simulink model "RexProblemSet2"  (R2020a)
settings: Solver=VariableStepAuto  StartTime=0.0  StopTime=10.0  RelTol=1e-3
undefined symbols (not defined in the file): gray
libraries: commutil2 x6, dspindex x4, visiontextngfix x2, visionsources x2
settings Model: Creator=23RexL  LastModifiedBy=23RexL

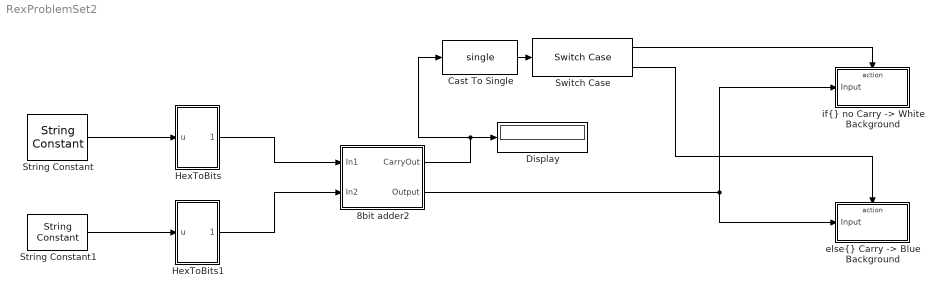
== system RexProblemSet2 ==
  8bit adder2 : Subsystem
  Cast To Single : DataTypeConversion  OutDataTypeStr=single
  Display : Display
  HexToBits : Subsystem
  HexToBits1 : Subsystem
  String Constant : StringConstant  String="\"FF\""
  String Constant1 : StringConstant  String="\"01\""
  Switch Case : SwitchCase  CaseConditions={0,1}  ShowDefaultCase=off  ZeroCross=off
  "else{} Carry -> Blue Background" : Subsystem  TreatAsAtomicUnit=on
  "if{} no Carry -> White Background" : Subsystem  TreatAsAtomicUnit=on
  wires:
  HexToBits/1(Out1) -> 8bit adder2/1(In1)
  String Constant1/1 -> HexToBits1/1(u)
  HexToBits1/1(Out1) -> 8bit adder2/2(In2)
  8bit adder2/1(CarryOut) -> Display/1, Cast To Single/1
  String Constant/1 -> HexToBits/1(u)
  Switch Case/2 -> "else{} Carry -> Blue Background"/Action
  Switch Case/1 -> "if{} no Carry -> White Background"/Action
  Cast To Single/1 -> Switch Case/1
  8bit adder2/2(Output) -> "if{} no Carry -> White Background"/1(Input), "else{} Carry -> Blue Background"/1(Input)

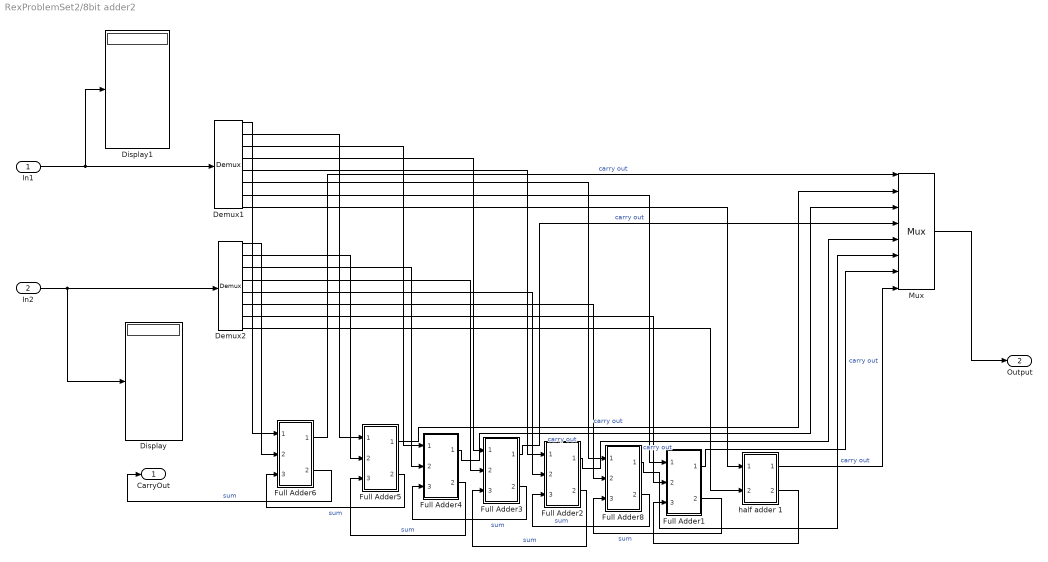
== system RexProblemSet2/8bit adder2 ==
  In1 : Inport
  In2 : Inport  Port=2
  Demux1 : Demux  Outputs=8
  Demux2 : Demux  Outputs=8
  Display : Display
  Display1 : Display
  Full Adder1 : Subsystem
  Full Adder2 : Subsystem
  Full Adder3 : Subsystem
  Full Adder4 : Subsystem
  Full Adder5 : Subsystem
  Full Adder6 : Subsystem
  Full Adder8 : Subsystem
  Mux : Mux  Inputs=8
  half adder 1 : Subsystem
  CarryOut : Outport
  Output : Outport  Port=2
  wires:
  Demux2/6 -> Full Adder8/2(Input1)
  Demux1/4 -> Full Adder3/1(Input)
  Demux2/4 -> Full Adder3/2(Input1)
  Demux2/8 -> half adder 1/2(Input2)
  Full Adder4/2(Output) -> Full Adder5/3(Input2)  "sum"
  Demux2/7 -> Full Adder1/2(Input1)
  Full Adder8/2(Output) -> Full Adder2/3(Input2)  "sum"
  Demux2/1 -> Full Adder6/2(Input1)
  Demux1/8 -> half adder 1/1(In1)
  Full Adder1/2(Output) -> Full Adder8/3(Input2)  "sum"
  In2/1 -> Display/1, Demux2/1
  Full Adder8/1(Output1) -> Mux/6  "carry out"
  Full Adder6/1(Output1) -> Mux/1  "carry out"
  Full Adder4/1(Output1) -> Mux/3  "carry out"
  Demux2/2 -> Full Adder5/2(Input1)
  Demux1/3 -> Full Adder4/1(Input)
  Full Adder5/1(Output1) -> Mux/2  "carry out"
  Demux2/3 -> Full Adder4/2(Input1)
  Full Adder3/1(Output1) -> Mux/4  "carry out"
  Full Adder3/2(Output) -> Full Adder4/3(Input2)  "sum"
  In1/1 -> Demux1/1, Display1/1
  Demux2/5 -> Full Adder2/2(Input1)
  Full Adder2/2(Output) -> Full Adder3/3(Input2)  "sum"
  half adder 1/2(Out2) -> Full Adder1/3(Input2)
  Full Adder2/1(Output1) -> Mux/5  "carry out"
  Demux1/5 -> Full Adder2/1(Input)
  Demux1/2 -> Full Adder5/1(Input)
  Full Adder5/2(Output) -> Full Adder6/3(Input2)  "sum"
  Demux1/1 -> Full Adder6/1(Input)
  Full Adder1/1(Output1) -> Mux/7  "carry out"
  half adder 1/1(Out1) -> Mux/8
  Demux1/7 -> Full Adder1/1(Input)
  Demux1/6 -> Full Adder8/1(Input)
  Mux/1 -> Output/1
  Full Adder6/2(Output) -> CarryOut/1  "sum"

== system RexProblemSet2/HexToBits ==
  u : Inport
  Integer to Bit Converter : commutil2/Integer to Bit Converter  nbits=8  signedInputValues=Unsigned  bitOrder=MSB first  outDtype=Inherit via internal rule
  MATLAB Function : MATLAB Function  TreatAsAtomicUnit=on
  Out1 : Outport
  wires:
  MATLAB Function/1(y) -> Integer to Bit Converter/1
  u/1 -> MATLAB Function/1(u)
  Integer to Bit Converter/1 -> Out1/1

== system RexProblemSet2/HexToBits1 ==
  u : Inport
  Integer to Bit Converter : commutil2/Integer to Bit Converter  nbits=8  signedInputValues=Unsigned  bitOrder=MSB first  outDtype=Inherit via internal rule
  MATLAB Function : MATLAB Function  TreatAsAtomicUnit=on
  Out1 : Outport
  wires:
  MATLAB Function/1(y) -> Integer to Bit Converter/1
  u/1 -> MATLAB Function/1(u)
  Integer to Bit Converter/1 -> Out1/1

== system RexProblemSet2/else{} Carry -> Blue Background ==
  Input : Inport
  Action Port : ActionPort  ActionPortLabel=case [ 1 ]:
  "else{} Carry -> Blue Background" : Subsystem
  wires:
  Input/1 -> "else{} Carry -> Blue Background"/1(Input1)

== system RexProblemSet2/if{} no Carry -> White Background ==
  Input : Inport
  Action Port : ActionPort  PropagateVarSize=During execution  ActionPortLabel=case [ 0 ]:
  "if{} no Carry -> White Background" : Subsystem
  wires:
  Input/1 -> "if{} no Carry -> White Background"/1(Input)

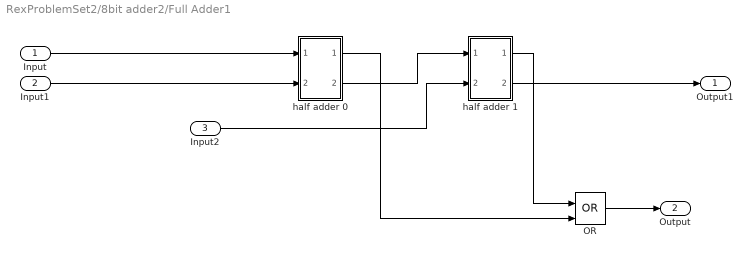
== system RexProblemSet2/8bit adder2/Full Adder1 ==
  Input : Inport
  Input1 : Inport  Port=2
  Input2 : Inport  Port=3
  OR : Logic  Operator=OR  IconShape=distinctive  AllPortsSameDT=off  OutDataTypeStr=boolean
  half adder 0 : Subsystem
  half adder 1 : Subsystem
  Output1 : Outport
  Output : Outport  Port=2
  wires:
  half adder 0/1(Out1) -> OR/2
  Input/1 -> half adder 0/1(Input)
  Input1/1 -> half adder 0/2(Input1)
  half adder 0/2(Out2) -> half adder 1/1(In1)
  half adder 1/1(Out1) -> OR/1
  OR/1 -> Output/1
  half adder 1/2(Output1) -> Output1/1
  Input2/1 -> half adder 1/2(Input2)

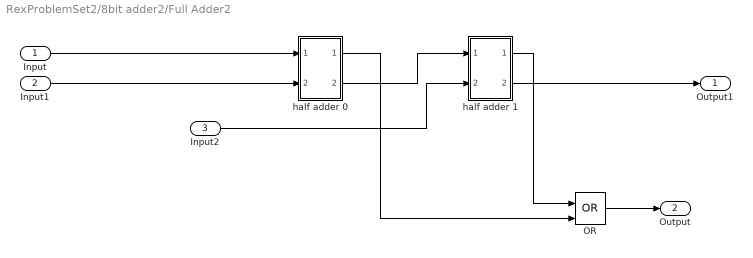
== system RexProblemSet2/8bit adder2/Full Adder2 ==
  Input : Inport
  Input1 : Inport  Port=2
  Input2 : Inport  Port=3
  OR : Logic  Operator=OR  IconShape=distinctive  AllPortsSameDT=off  OutDataTypeStr=boolean
  half adder 0 : Subsystem
  half adder 1 : Subsystem
  Output1 : Outport
  Output : Outport  Port=2
  wires:
  half adder 0/1(Out1) -> OR/2
  Input/1 -> half adder 0/1(Input)
  Input1/1 -> half adder 0/2(Input1)
  half adder 0/2(Out2) -> half adder 1/1(In1)
  half adder 1/1(Out1) -> OR/1
  OR/1 -> Output/1
  half adder 1/2(Output1) -> Output1/1
  Input2/1 -> half adder 1/2(Input2)

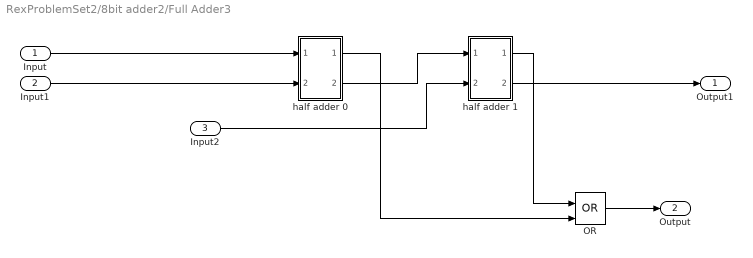
== system RexProblemSet2/8bit adder2/Full Adder3 ==
  Input : Inport
  Input1 : Inport  Port=2
  Input2 : Inport  Port=3
  OR : Logic  Operator=OR  IconShape=distinctive  AllPortsSameDT=off  OutDataTypeStr=boolean
  half adder 0 : Subsystem
  half adder 1 : Subsystem
  Output1 : Outport
  Output : Outport  Port=2
  wires:
  half adder 0/1(Out1) -> OR/2
  Input/1 -> half adder 0/1(Input)
  Input1/1 -> half adder 0/2(Input1)
  half adder 0/2(Out2) -> half adder 1/1(In1)
  half adder 1/1(Out1) -> OR/1
  OR/1 -> Output/1
  half adder 1/2(Output1) -> Output1/1
  Input2/1 -> half adder 1/2(Input2)

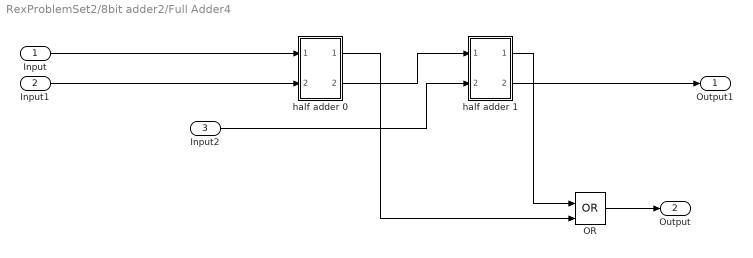
== system RexProblemSet2/8bit adder2/Full Adder4 ==
  Input : Inport
  Input1 : Inport  Port=2
  Input2 : Inport  Port=3
  OR : Logic  Operator=OR  IconShape=distinctive  AllPortsSameDT=off  OutDataTypeStr=boolean
  half adder 0 : Subsystem
  half adder 1 : Subsystem
  Output1 : Outport
  Output : Outport  Port=2
  wires:
  half adder 0/1(Out1) -> OR/2
  Input/1 -> half adder 0/1(Input)
  Input1/1 -> half adder 0/2(Input1)
  half adder 0/2(Out2) -> half adder 1/1(In1)
  half adder 1/1(Out1) -> OR/1
  OR/1 -> Output/1
  half adder 1/2(Output1) -> Output1/1
  Input2/1 -> half adder 1/2(Input2)

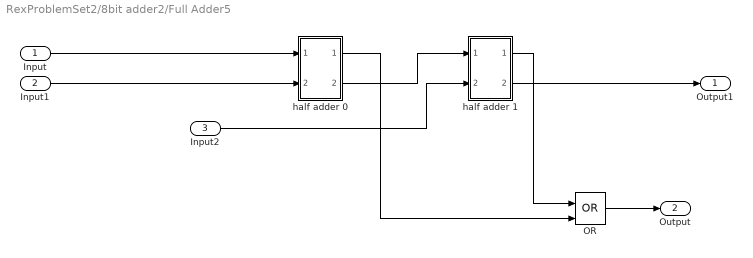
== system RexProblemSet2/8bit adder2/Full Adder5 ==
  Input : Inport
  Input1 : Inport  Port=2
  Input2 : Inport  Port=3
  OR : Logic  Operator=OR  IconShape=distinctive  AllPortsSameDT=off  OutDataTypeStr=boolean
  half adder 0 : Subsystem
  half adder 1 : Subsystem
  Output1 : Outport
  Output : Outport  Port=2
  wires:
  half adder 0/1(Out1) -> OR/2
  Input/1 -> half adder 0/1(Input)
  Input1/1 -> half adder 0/2(Input1)
  half adder 0/2(Out2) -> half adder 1/1(In1)
  half adder 1/1(Out1) -> OR/1
  OR/1 -> Output/1
  half adder 1/2(Output1) -> Output1/1
  Input2/1 -> half adder 1/2(Input2)

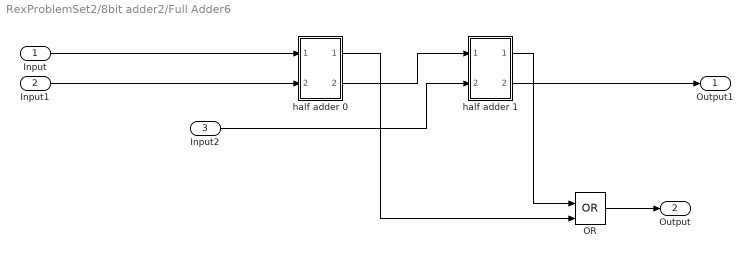
== system RexProblemSet2/8bit adder2/Full Adder6 ==
  Input : Inport
  Input1 : Inport  Port=2
  Input2 : Inport  Port=3
  OR : Logic  Operator=OR  IconShape=distinctive  AllPortsSameDT=off  OutDataTypeStr=boolean
  half adder 0 : Subsystem
  half adder 1 : Subsystem
  Output1 : Outport
  Output : Outport  Port=2
  wires:
  half adder 0/1(Out1) -> OR/2
  Input/1 -> half adder 0/1(Input)
  Input1/1 -> half adder 0/2(Input1)
  half adder 0/2(Out2) -> half adder 1/1(In1)
  half adder 1/1(Out1) -> OR/1
  OR/1 -> Output/1
  half adder 1/2(Output1) -> Output1/1
  Input2/1 -> half adder 1/2(Input2)

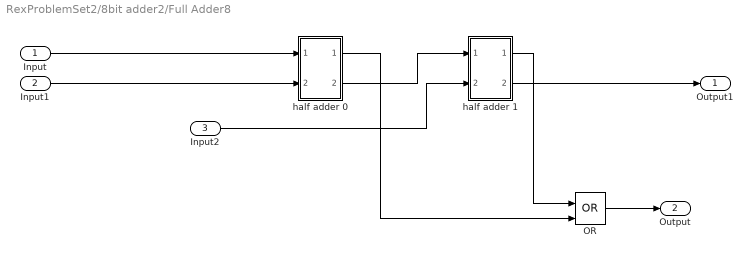
== system RexProblemSet2/8bit adder2/Full Adder8 ==
  Input : Inport
  Input1 : Inport  Port=2
  Input2 : Inport  Port=3
  OR : Logic  Operator=OR  IconShape=distinctive  AllPortsSameDT=off  OutDataTypeStr=boolean
  half adder 0 : Subsystem
  half adder 1 : Subsystem
  Output1 : Outport
  Output : Outport  Port=2
  wires:
  half adder 0/1(Out1) -> OR/2
  Input/1 -> half adder 0/1(Input)
  Input1/1 -> half adder 0/2(Input1)
  half adder 0/2(Out2) -> half adder 1/1(In1)
  half adder 1/1(Out1) -> OR/1
  OR/1 -> Output/1
  half adder 1/2(Output1) -> Output1/1
  Input2/1 -> half adder 1/2(Input2)

== system RexProblemSet2/8bit adder2/half adder 1 ==
  In1 : Inport
  Input2 : Inport  Port=2
  NAND : Logic  IconShape=distinctive  AllPortsSameDT=off  OutDataTypeStr=boolean
  XOR : Logic  Operator=XOR  IconShape=distinctive  AllPortsSameDT=off  OutDataTypeStr=boolean
  Out1 : Outport
  Out2 : Outport  Port=2
  wires:
  Input2/1 -> NAND/2, XOR/2
  In1/1 -> NAND/1, XOR/1
  NAND/1 -> Out2/1
  XOR/1 -> Out1/1

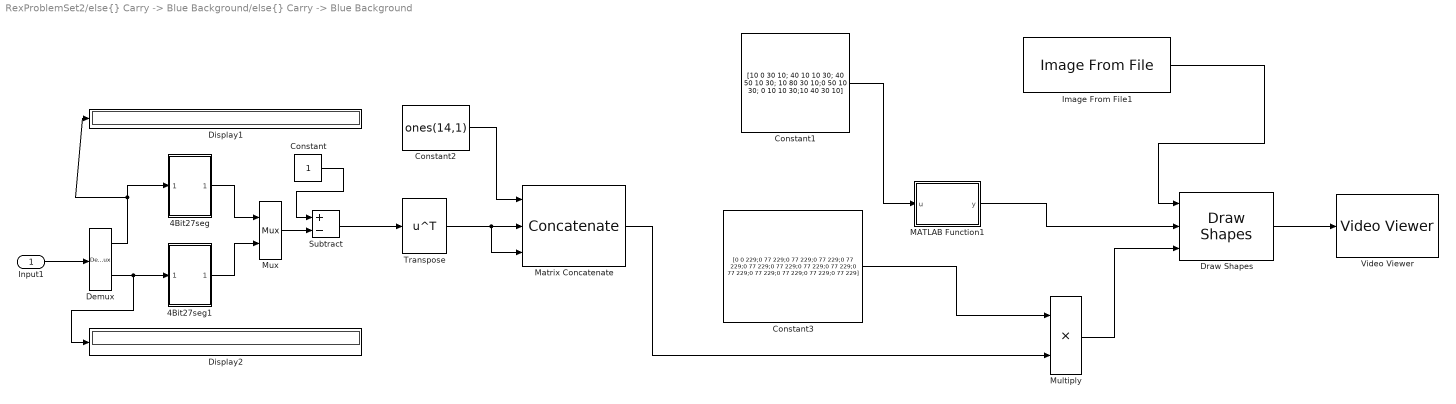
== system RexProblemSet2/else{} Carry -> Blue Background/else{} Carry -> Blue Background ==
  Input1 : Inport
  4Bit27seg : Subsystem
  4Bit27seg1 : Subsystem
  Constant : Constant
  Constant1 : Constant  Value="[10 0  30 10; 40 10 10 30; 40 50 10 30; 10 80 30 10;0 50 10 30; 0 10 10 30;10 40 30 10]"  VectorParams1D=off
  Constant2 : Constant  Value=ones(14,1)
  Constant3 : Constant  Value=[0 0 229;0 77 229;0 77 229;0 77 229;0 77 229;0 77 229;0 77 229;0 77 229;0 77 229;0 77 229;0 77 229;0 77 229;0 77 229;0 77 229]  VectorParams1D=off
  Demux : Demux  Outputs=2
  Display1 : Display
  Display2 : Display
  Draw Shapes : visiontextngfix/Draw Shapes  shape=Rectangles  fill=on  lineWidth=1  fillClrSource=Input port  display=Black  intensity=200  color=[200 255 100]  opacity=0.6  viewport=Entire image  antialiasing=off  inType=Obsolete  imagePorts=One multidimensional signal  roundingMode=Floor  overflowMode=off  memoryMode=Specify word length  memoryWordLength=16  prodOutputMode=Binary point scaling  prodOutputWordLength=32  prodOutputFracLength=14  memoryFracLength=14
  Image From File1 : visionsources/Image From File  Tag=vipblks_nd  FileName=C:\Users\23rexl\Desktop\Rex ProblemSet 2\BlueBackground.jpg  Ts=inf  imagePorts=One multidimensional signal  OutPortLabels=R|G|B  ImageDataType=double  sdImageDataType=uint(8)  Signed=on  WordLength=16  FractionLengthMode=User-defined  FractionLength=15
      link override Constant1: Value=ImageValue
  MATLAB Function1 : MATLAB Function  TreatAsAtomicUnit=on
  Matrix Concatenate : Concatenate  NumInputs=3  Mode=Multidimensional array  ConcatenateDimension=2
  Multiply : Product
  Mux : Mux  Inputs=2
  Subtract : Sum  Inputs=+-
  Transpose : Math  Operator=transpose  SaturateOnIntegerOverflow=on
  Video Viewer : VideoViewer  colormapValue=gray(256)  FigPos=[810.6 762 480.8 371.2]
  wires:
  Mux/1 -> Subtract/2
  Constant2/1 -> Matrix Concatenate/1
  Matrix Concatenate/1 -> Multiply/2
  Multiply/1 -> Draw Shapes/3
  Constant3/1 -> Multiply/1
  Demux/1 -> 4Bit27seg/1(Input), Display1/1
  Subtract/1 -> Transpose/1
  Draw Shapes/1 -> Video Viewer/1
  4Bit27seg1/1(Output) -> Mux/2
  Demux/2 -> Display2/1, 4Bit27seg1/1(Input)
  Constant1/1 -> MATLAB Function1/1(u)
  4Bit27seg/1(Output) -> Mux/1
  Constant/1 -> Subtract/1
  Image From File1/1 -> Draw Shapes/1
  MATLAB Function1/1(y) -> Draw Shapes/2
  Transpose/1 -> Matrix Concatenate/3, Matrix Concatenate/2
  Input1/1 -> Demux/1

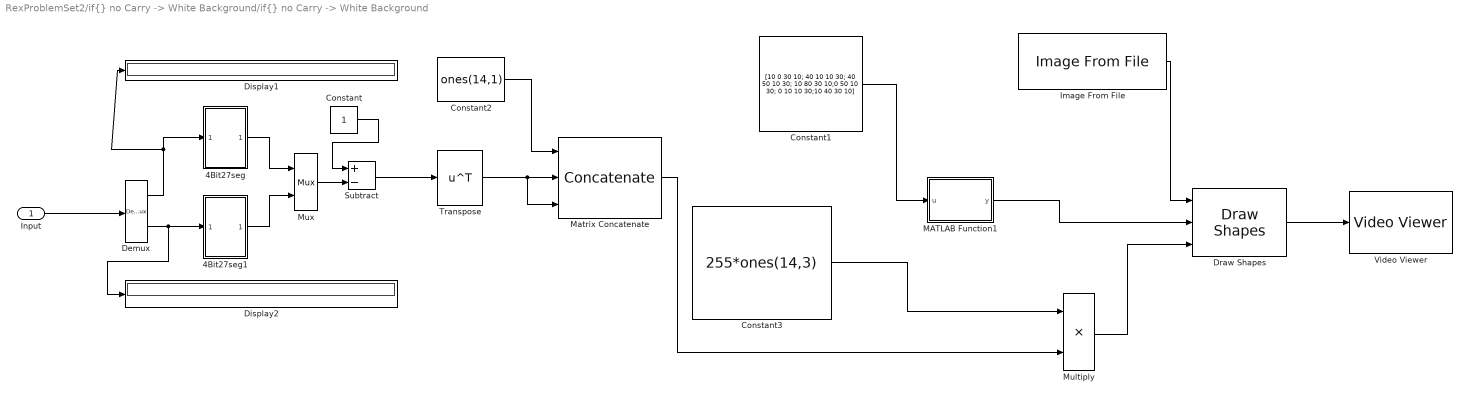
== system RexProblemSet2/if{} no Carry -> White Background/if{} no Carry -> White Background ==
  Input : Inport
  4Bit27seg : Subsystem
  4Bit27seg1 : Subsystem
  Constant : Constant
  Constant1 : Constant  Value="[10 0  30 10; 40 10 10 30; 40 50 10 30; 10 80 30 10;0 50 10 30; 0 10 10 30;10 40 30 10]"  VectorParams1D=off
  Constant2 : Constant  Value=ones(14,1)
  Constant3 : Constant  Value=255*ones(14,3)
  Demux : Demux  Outputs=2
  Display1 : Display
  Display2 : Display
  Draw Shapes : visiontextngfix/Draw Shapes  shape=Rectangles  fill=on  lineWidth=1  fillClrSource=Input port  display=Black  intensity=200  color=[200 255 100]  opacity=0.6  viewport=Entire image  antialiasing=off  inType=Obsolete  imagePorts=One multidimensional signal  roundingMode=Floor  overflowMode=off  memoryMode=Specify word length  memoryWordLength=16  prodOutputMode=Binary point scaling  prodOutputWordLength=32  prodOutputFracLength=14  memoryFracLength=14
  Image From File : visionsources/Image From File  Tag=vipblks_nd  FileName=C:\Users\23rexl\Desktop\Rex ProblemSet 2\WhiteBackground (1).png  Ts=inf  imagePorts=One multidimensional signal  OutPortLabels=R|G|B  ImageDataType=double  sdImageDataType=uint(8)  Signed=on  WordLength=16  FractionLengthMode=User-defined  FractionLength=15
      link override Constant1: Value=ImageValue
  MATLAB Function1 : MATLAB Function  TreatAsAtomicUnit=on
  Matrix Concatenate : Concatenate  NumInputs=3  Mode=Multidimensional array  ConcatenateDimension=2
  Multiply : Product
  Mux : Mux  Inputs=2
  Subtract : Sum  Inputs=+-
  Transpose : Math  Operator=transpose  SaturateOnIntegerOverflow=on
  Video Viewer : VideoViewer  colormapValue=gray(256)  FigPos=[117.8 924.4 648 477.6]
  wires:
  Mux/1 -> Subtract/2
  Constant2/1 -> Matrix Concatenate/1
  Matrix Concatenate/1 -> Multiply/2
  Multiply/1 -> Draw Shapes/3
  Constant3/1 -> Multiply/1
  Demux/1 -> 4Bit27seg/1(Input), Display1/1
  Subtract/1 -> Transpose/1
  Draw Shapes/1 -> Video Viewer/1
  4Bit27seg1/1(Output) -> Mux/2
  Demux/2 -> Display2/1, 4Bit27seg1/1(Input)
  Constant1/1 -> MATLAB Function1/1(u)
  4Bit27seg/1(Output) -> Mux/1
  Constant/1 -> Subtract/1
  Image From File/1 -> Draw Shapes/1
  MATLAB Function1/1(y) -> Draw Shapes/2
  Transpose/1 -> Matrix Concatenate/3, Matrix Concatenate/2
  Input/1 -> Demux/1

== system RexProblemSet2/8bit adder2/Full Adder1/half adder 0 ==
  Input : Inport
  Input1 : Inport  Port=2
  XOR : Logic  Operator=XOR  IconShape=distinctive  AllPortsSameDT=off  OutDataTypeStr=boolean
  and : Logic  IconShape=distinctive  AllPortsSameDT=off  OutDataTypeStr=boolean
  Out1 : Outport
  Out2 : Outport  Port=2
  wires:
  Input1/1 -> and/2, XOR/2
  Input/1 -> and/1, XOR/1
  and/1 -> Out1/1
  XOR/1 -> Out2/1

== system RexProblemSet2/8bit adder2/Full Adder1/half adder 1 ==
  In1 : Inport
  Input2 : Inport  Port=2
  AND : Logic  IconShape=distinctive  AllPortsSameDT=off  OutDataTypeStr=boolean
  XOR : Logic  Operator=XOR  IconShape=distinctive  AllPortsSameDT=off  OutDataTypeStr=boolean
  Out1 : Outport
  Output1 : Outport  Port=2
  wires:
  Input2/1 -> AND/2, XOR/2
  In1/1 -> AND/1, XOR/1
  AND/1 -> Out1/1
  XOR/1 -> Output1/1

== system RexProblemSet2/8bit adder2/Full Adder2/half adder 0 ==
  Input : Inport
  Input1 : Inport  Port=2
  XOR : Logic  Operator=XOR  IconShape=distinctive  AllPortsSameDT=off  OutDataTypeStr=boolean
  and : Logic  IconShape=distinctive  AllPortsSameDT=off  OutDataTypeStr=boolean
  Out1 : Outport
  Out2 : Outport  Port=2
  wires:
  Input1/1 -> and/2, XOR/2
  Input/1 -> and/1, XOR/1
  and/1 -> Out1/1
  XOR/1 -> Out2/1

== system RexProblemSet2/8bit adder2/Full Adder2/half adder 1 ==
  In1 : Inport
  Input2 : Inport  Port=2
  AND : Logic  IconShape=distinctive  AllPortsSameDT=off  OutDataTypeStr=boolean
  XOR : Logic  Operator=XOR  IconShape=distinctive  AllPortsSameDT=off  OutDataTypeStr=boolean
  Out1 : Outport
  Output1 : Outport  Port=2
  wires:
  Input2/1 -> AND/2, XOR/2
  In1/1 -> AND/1, XOR/1
  AND/1 -> Out1/1
  XOR/1 -> Output1/1

== system RexProblemSet2/8bit adder2/Full Adder3/half adder 0 ==
  Input : Inport
  Input1 : Inport  Port=2
  XOR : Logic  Operator=XOR  IconShape=distinctive  AllPortsSameDT=off  OutDataTypeStr=boolean
  and : Logic  IconShape=distinctive  AllPortsSameDT=off  OutDataTypeStr=boolean
  Out1 : Outport
  Out2 : Outport  Port=2
  wires:
  Input1/1 -> and/2, XOR/2
  Input/1 -> and/1, XOR/1
  and/1 -> Out1/1
  XOR/1 -> Out2/1

== system RexProblemSet2/8bit adder2/Full Adder3/half adder 1 ==
  In1 : Inport
  Input2 : Inport  Port=2
  AND : Logic  IconShape=distinctive  AllPortsSameDT=off  OutDataTypeStr=boolean
  XOR : Logic  Operator=XOR  IconShape=distinctive  AllPortsSameDT=off  OutDataTypeStr=boolean
  Out1 : Outport
  Output1 : Outport  Port=2
  wires:
  Input2/1 -> AND/2, XOR/2
  In1/1 -> AND/1, XOR/1
  AND/1 -> Out1/1
  XOR/1 -> Output1/1

== system RexProblemSet2/8bit adder2/Full Adder4/half adder 0 ==
  Input : Inport
  Input1 : Inport  Port=2
  XOR : Logic  Operator=XOR  IconShape=distinctive  AllPortsSameDT=off  OutDataTypeStr=boolean
  and : Logic  IconShape=distinctive  AllPortsSameDT=off  OutDataTypeStr=boolean
  Out1 : Outport
  Out2 : Outport  Port=2
  wires:
  Input1/1 -> and/2, XOR/2
  Input/1 -> and/1, XOR/1
  and/1 -> Out1/1
  XOR/1 -> Out2/1

== system RexProblemSet2/8bit adder2/Full Adder4/half adder 1 ==
  In1 : Inport
  Input2 : Inport  Port=2
  AND : Logic  IconShape=distinctive  AllPortsSameDT=off  OutDataTypeStr=boolean
  XOR : Logic  Operator=XOR  IconShape=distinctive  AllPortsSameDT=off  OutDataTypeStr=boolean
  Out1 : Outport
  Output1 : Outport  Port=2
  wires:
  Input2/1 -> AND/2, XOR/2
  In1/1 -> AND/1, XOR/1
  AND/1 -> Out1/1
  XOR/1 -> Output1/1

== system RexProblemSet2/8bit adder2/Full Adder5/half adder 0 ==
  Input : Inport
  Input1 : Inport  Port=2
  XOR : Logic  Operator=XOR  IconShape=distinctive  AllPortsSameDT=off  OutDataTypeStr=boolean
  and : Logic  IconShape=distinctive  AllPortsSameDT=off  OutDataTypeStr=boolean
  Out1 : Outport
  Out2 : Outport  Port=2
  wires:
  Input1/1 -> and/2, XOR/2
  Input/1 -> and/1, XOR/1
  and/1 -> Out1/1
  XOR/1 -> Out2/1

== system RexProblemSet2/8bit adder2/Full Adder5/half adder 1 ==
  In1 : Inport
  Input2 : Inport  Port=2
  AND : Logic  IconShape=distinctive  AllPortsSameDT=off  OutDataTypeStr=boolean
  XOR : Logic  Operator=XOR  IconShape=distinctive  AllPortsSameDT=off  OutDataTypeStr=boolean
  Out1 : Outport
  Output1 : Outport  Port=2
  wires:
  Input2/1 -> AND/2, XOR/2
  In1/1 -> AND/1, XOR/1
  AND/1 -> Out1/1
  XOR/1 -> Output1/1

== system RexProblemSet2/8bit adder2/Full Adder6/half adder 0 ==
  Input : Inport
  Input1 : Inport  Port=2
  XOR : Logic  Operator=XOR  IconShape=distinctive  AllPortsSameDT=off  OutDataTypeStr=boolean
  and : Logic  IconShape=distinctive  AllPortsSameDT=off  OutDataTypeStr=boolean
  Out1 : Outport
  Out2 : Outport  Port=2
  wires:
  Input1/1 -> and/2, XOR/2
  Input/1 -> and/1, XOR/1
  and/1 -> Out1/1
  XOR/1 -> Out2/1

== system RexProblemSet2/8bit adder2/Full Adder6/half adder 1 ==
  In1 : Inport
  Input2 : Inport  Port=2
  AND : Logic  IconShape=distinctive  AllPortsSameDT=off  OutDataTypeStr=boolean
  XOR : Logic  Operator=XOR  IconShape=distinctive  AllPortsSameDT=off  OutDataTypeStr=boolean
  Out1 : Outport
  Output1 : Outport  Port=2
  wires:
  Input2/1 -> AND/2, XOR/2
  In1/1 -> AND/1, XOR/1
  AND/1 -> Out1/1
  XOR/1 -> Output1/1

== system RexProblemSet2/8bit adder2/Full Adder8/half adder 0 ==
  Input : Inport
  Input1 : Inport  Port=2
  XOR : Logic  Operator=XOR  IconShape=distinctive  AllPortsSameDT=off  OutDataTypeStr=boolean
  and : Logic  IconShape=distinctive  AllPortsSameDT=off  OutDataTypeStr=boolean
  Out1 : Outport
  Out2 : Outport  Port=2
  wires:
  Input1/1 -> and/2, XOR/2
  Input/1 -> and/1, XOR/1
  and/1 -> Out1/1
  XOR/1 -> Out2/1

== system RexProblemSet2/8bit adder2/Full Adder8/half adder 1 ==
  In1 : Inport
  Input2 : Inport  Port=2
  AND : Logic  IconShape=distinctive  AllPortsSameDT=off  OutDataTypeStr=boolean
  XOR : Logic  Operator=XOR  IconShape=distinctive  AllPortsSameDT=off  OutDataTypeStr=boolean
  Out1 : Outport
  Output1 : Outport  Port=2
  wires:
  Input2/1 -> AND/2, XOR/2
  In1/1 -> AND/1, XOR/1
  AND/1 -> Out1/1
  XOR/1 -> Output1/1

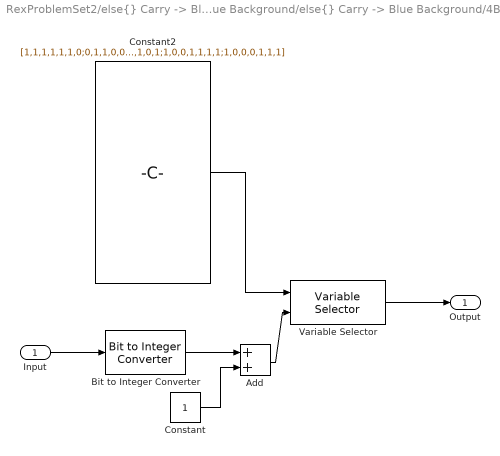
== system RexProblemSet2/else{} Carry -> Blue Background/else{} Carry -> Blue Background/4Bit27seg ==
  Input : Inport
  Add : Sum
  Bit to Integer Converter : commutil2/Bit to Integer Converter  nbits=4  bitOrder=MSB first  signedOutputValues=Unsigned  outDtype=Inherit via internal rule  outDtypeSigned=Inherit via internal rule
  Constant : Constant
  Constant2 : Constant  Value=[1,1,1,1,1,1,0;0,1,1,0,0,0,0;1,1,0,1,1,0,1;1,1,1,1,0,0,1;0,1,1,0,0,1,1;1,0,1,1,0,1,1;1,0,1,1,1,1,1;1,1,1,0,0,0,0;1,1,1,1,1,1,1;1,1,1,1,0,1,1;1,1,1,0,1,1,1;0,0,1,1,1,1,1;1,0,0,1,1,1,0;0,1,1,1,1,0,1;1,0,0,1,1,1,1;1,0,0,0,1,1,1]
  Variable Selector : dspindex/Variable Selector  NumInputs=1  rowsOrCols=Rows  IdxMode=Variable  Elements=[1 3]  ZerOneIdxMode=One-based  errmode=Clip Index  FillMode=on  FillValues=0
  Output : Outport
  wires:
  Bit to Integer Converter/1 -> Add/1
  Constant/1 -> Add/2
  Add/1 -> Variable Selector/2
  Constant2/1 -> Variable Selector/1
  Variable Selector/1 -> Output/1
  Input/1 -> Bit to Integer Converter/1

== system RexProblemSet2/else{} Carry -> Blue Background/else{} Carry -> Blue Background/4Bit27seg1 ==
  Input : Inport
  Add : Sum
  Bit to Integer Converter : commutil2/Bit to Integer Converter  nbits=4  bitOrder=MSB first  signedOutputValues=Unsigned  outDtype=Inherit via internal rule  outDtypeSigned=Inherit via internal rule
  Constant : Constant
  Constant2 : Constant  Value=[1,1,1,1,1,1,0;0,1,1,0,0,0,0;1,1,0,1,1,0,1;1,1,1,1,0,0,1;0,1,1,0,0,1,1;1,0,1,1,0,1,1;1,0,1,1,1,1,1;1,1,1,0,0,0,0;1,1,1,1,1,1,1;1,1,1,1,0,1,1;1,1,1,0,1,1,1;0,0,1,1,1,1,1;1,0,0,1,1,1,0;0,1,1,1,1,0,1;1,0,0,1,1,1,1;1,0,0,0,1,1,1]
  Variable Selector : dspindex/Variable Selector  NumInputs=1  rowsOrCols=Rows  IdxMode=Variable  Elements=[1 3]  ZerOneIdxMode=One-based  errmode=Clip Index  FillMode=on  FillValues=0
  Output : Outport
  wires:
  Bit to Integer Converter/1 -> Add/1
  Constant/1 -> Add/2
  Add/1 -> Variable Selector/2
  Constant2/1 -> Variable Selector/1
  Variable Selector/1 -> Output/1
  Input/1 -> Bit to Integer Converter/1

== system RexProblemSet2/if{} no Carry -> White Background/if{} no Carry -> White Background/4Bit27seg ==
  Input : Inport
  Add : Sum
  Bit to Integer Converter : commutil2/Bit to Integer Converter  nbits=4  bitOrder=MSB first  signedOutputValues=Unsigned  outDtype=Inherit via internal rule  outDtypeSigned=Inherit via internal rule
  Constant : Constant
  Constant2 : Constant  Value=[1,1,1,1,1,1,0;0,1,1,0,0,0,0;1,1,0,1,1,0,1;1,1,1,1,0,0,1;0,1,1,0,0,1,1;1,0,1,1,0,1,1;1,0,1,1,1,1,1;1,1,1,0,0,0,0;1,1,1,1,1,1,1;1,1,1,1,0,1,1;1,1,1,0,1,1,1;0,0,1,1,1,1,1;1,0,0,1,1,1,0;0,1,1,1,1,0,1;1,0,0,1,1,1,1;1,0,0,0,1,1,1]
  Variable Selector : dspindex/Variable Selector  NumInputs=1  rowsOrCols=Rows  IdxMode=Variable  Elements=[1 3]  ZerOneIdxMode=One-based  errmode=Clip Index  FillMode=on  FillValues=0
  Output : Outport
  wires:
  Bit to Integer Converter/1 -> Add/1
  Constant/1 -> Add/2
  Add/1 -> Variable Selector/2
  Constant2/1 -> Variable Selector/1
  Variable Selector/1 -> Output/1
  Input/1 -> Bit to Integer Converter/1

== system RexProblemSet2/if{} no Carry -> White Background/if{} no Carry -> White Background/4Bit27seg1 ==
  Input : Inport
  Add : Sum
  Bit to Integer Converter : commutil2/Bit to Integer Converter  nbits=4  bitOrder=MSB first  signedOutputValues=Unsigned  outDtype=Inherit via internal rule  outDtypeSigned=Inherit via internal rule
  Constant : Constant
  Constant2 : Constant  Value=[1,1,1,1,1,1,0;0,1,1,0,0,0,0;1,1,0,1,1,0,1;1,1,1,1,0,0,1;0,1,1,0,0,1,1;1,0,1,1,0,1,1;1,0,1,1,1,1,1;1,1,1,0,0,0,0;1,1,1,1,1,1,1;1,1,1,1,0,1,1;1,1,1,0,1,1,1;0,0,1,1,1,1,1;1,0,0,1,1,1,0;0,1,1,1,1,0,1;1,0,0,1,1,1,1;1,0,0,0,1,1,1]
  Variable Selector : dspindex/Variable Selector  NumInputs=1  rowsOrCols=Rows  IdxMode=Variable  Elements=[1 3]  ZerOneIdxMode=One-based  errmode=Clip Index  FillMode=on  FillValues=0
  Output : Outport
  wires:
  Bit to Integer Converter/1 -> Add/1
  Constant/1 -> Add/2
  Add/1 -> Variable Selector/2
  Constant2/1 -> Variable Selector/1
  Variable Selector/1 -> Output/1
  Input/1 -> Bit to Integer Converter/1

== matlab function RexProblemSet2/HexToBits/MATLAB Function ==
  data: u input; y output
function y = hexTodec(u)
y=0;
y = hex2dec(u);

== matlab function RexProblemSet2/HexToBits1/MATLAB Function ==
  data: u input; y output
function y = hexTodec(u)
y=0;
y = hex2dec(u);

== matlab function RexProblemSet2/else{} Carry -> Blue Background/else{} Carry -> Blue Background/MATLAB Function1 ==
  data: u input; y output
function y = fcn(u)
v = repmat([60 0 0 0],7,1)
v = u+v;
y = [u;v];

== matlab function RexProblemSet2/if{} no Carry -> White Background/if{} no Carry -> White Background/MATLAB Function1 ==
  data: u input; y output
function y = fcn(u)
v = repmat([60 0 0 0],7,1)
v = u+v;
y = [u;v];
